simulink model "Non_isolated_Buck_Boost_Converter_w_NonIdealities"  (R2021a)
settings: Solver=VariableStepAuto  StartTime=0.0  StopTime=0.1  RelTol=1e-3
libraries: spsSeriesRLCBranchLib x5, spsCurrentMeasurementLib x4, spsVoltageMeasurementLib x3, spsDiodeLib x1, spsMosfetLib x1, spsDCVoltageSourceLib x1, spspowerguiLib x1
settings Model: Creator=EREN-PC  LastModifiedBy=EREN-PC

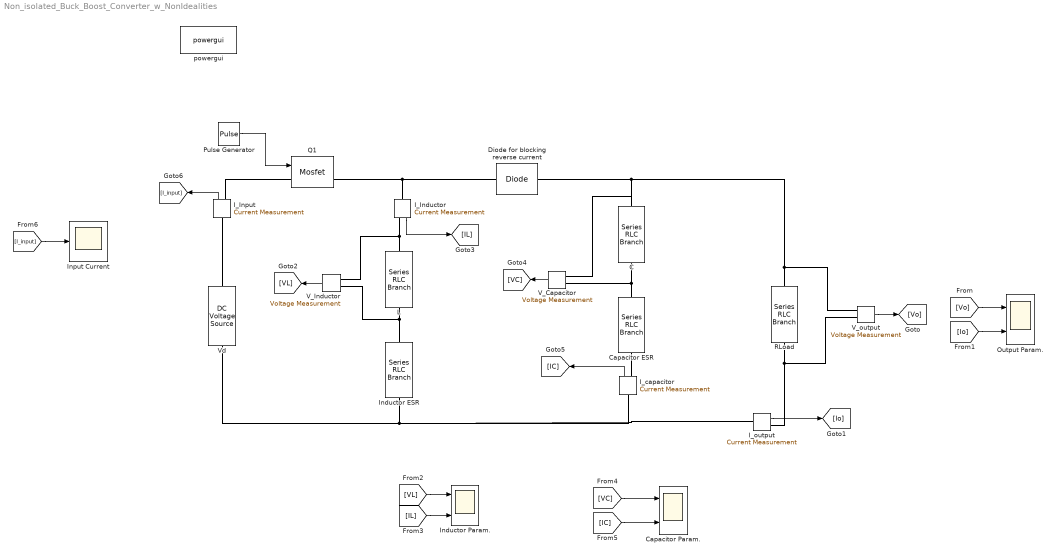
== system Non_isolated_Buck_Boost_Converter_w_NonIdealities ==
  C : spsSeriesRLCBranchLib/Series RLC Branch  LConnTagsString=__new0  RConnTagsString=__new0  BranchType=C  Resistance=1  Inductance=1e-3  SetiL0=off  InitialCurrent=0  Capacitance=1e-3  Setx0=off  InitialVoltage=0  Measurements=None
  Capacitor ESR : spsSeriesRLCBranchLib/Series RLC Branch  LConnTagsString=__new0  RConnTagsString=__new0  BranchType=R  Resistance=12e-3  Inductance=1e-3  SetiL0=off  InitialCurrent=0  Capacitance=1e-6  Setx0=off  InitialVoltage=0  Measurements=None
  Capacitor Param. : Scope  NumInputPorts=2
  Diode for blocking reverse current : spsDiodeLib/Diode  Ron=0.001  Lon=0  Vf=0.45  IC=0  UseSnubber=0  Rs=500  Cs=250e-9  Measurements=off
  I_Inductor : spsCurrentMeasurementLib/Current Measurement  PhasorSimulation=off  OutputType=Complex  PSBequivalent=0
  I_Input : spsCurrentMeasurementLib/Current Measurement  PhasorSimulation=off  OutputType=Complex  PSBequivalent=0
  I_capacitor : spsCurrentMeasurementLib/Current Measurement  PhasorSimulation=off  OutputType=Complex  PSBequivalent=0
  I_output : spsCurrentMeasurementLib/Current Measurement  PhasorSimulation=off  OutputType=Complex  PSBequivalent=0
  Inductor ESR : spsSeriesRLCBranchLib/Series RLC Branch  LConnTagsString=__new0  RConnTagsString=__new0  BranchType=R  Resistance=0.494  Inductance=1e-3  SetiL0=off  InitialCurrent=0  Capacitance=1e-6  Setx0=off  InitialVoltage=0  Measurements=None
  Inductor Param. : Scope  NumInputPorts=2
  Input Current : Scope
  L : spsSeriesRLCBranchLib/Series RLC Branch  LConnTagsString=__new0  RConnTagsString=__new0  BranchType=L  Resistance=0.494  Inductance=2.2e-3  SetiL0=off  InitialCurrent=0  Capacitance=1e-6  Setx0=off  InitialVoltage=0  Measurements=None
  Output Param. : Scope  NumInputPorts=2
  Pulse Generator : DiscretePulseGenerator  PulseType=Time based  Period=20e-6  PulseWidth=52
  Q1 : spsMosfetLib/Mosfet  Ron=60e-3  Lon=0  Rd=25e-3  Vfd=0  IC=0  Rs=1e5  Cs=inf  Measurements=on
  RLoad : spsSeriesRLCBranchLib/Series RLC Branch  LConnTagsString=__new0  RConnTagsString=__new0  BranchType=R  Resistance=6  Inductance=1e-3  SetiL0=off  InitialCurrent=0  Capacitance=1e-6  Setx0=off  InitialVoltage=0  Measurements=None
  V_Capacitor : spsVoltageMeasurementLib/Voltage Measurement  PhasorSimulation=off  OutputType=Complex  PSBequivalent=0
  V_Inductor : spsVoltageMeasurementLib/Voltage Measurement  PhasorSimulation=off  OutputType=Complex  PSBequivalent=0
  V_output : spsVoltageMeasurementLib/Voltage Measurement  PhasorSimulation=off  OutputType=Complex  PSBequivalent=0
  Vd : spsDCVoltageSourceLib/DC Voltage Source  Amplitude=16  Measurements=None
  powergui : spspowerguiLib/powergui  Priority=1  SimulationMode=Continuous  SampleTime=50e-6  frequency=60  Iterations=50  frequencyindice=0  Pbase=100e6  ErrMax=1e-4  UnitsV=kV  UnitsW=MW  buscounter=0  FunctionMessages=off  echomessages=off  EnableUseOfTLC=off  CurrentSourceSwitches=off  DisableSnubberDevices=off  DisableRonSwitches=off  DisableVfSwitches=off  DisplayEquations=off  AutomaticDiscreteSolvers=off  SolverType=Tustin/Backward Euler (TBE)  Interpol=off  ExternalGateDelay=off  methode=off  Ts=100  x0status=blocks  SPID=on  SwTol=0  HookPort=off  NonlinearTolerance=1e-4  nMaxIteration=100  ContinueOnMaxIteration=off  RestoreLinks=warning  ResistiveCurrentMeasurement=off  Frange=[0:2:500]  Ylog=off  Xlog=on  ShowGrid=off  save=off  variable=ZData  structure=0  ZoomFFT=off  StartTime=0.0  cycles=1  DisplayStyle=1  fundamental=60  FreqAxis=off  MaxFrequency=1000  frequencyindicesteady=1  RmsSteady=1  display=off
  wires:
  V_output/1 -> [Vo]
  [Vo] -> Output Param./1
  I_output/1 -> [Io]
  [Io] -> Output Param./2
  V_Inductor/1 -> [VL]
  [VL] -> Inductor Param./1
  I_Inductor/1 -> [IL]
  [IL] -> Inductor Param./2
  V_Capacitor/1 -> [VC]
  [VC] -> Capacitor Param./1
  I_capacitor/1 -> [IC]
  [IC] -> Capacitor Param./2
  Pulse Generator/1 -> Q1/1
  I_Input/1 -> [I_input]
  [I_input] -> Input Current/1
  connections:
  Inductor ESR/RConn1 -- I_capacitor/LConn1 -- I_output/LConn1 -- Vd/LConn1
  Q1/RConn1 -- I_Inductor/LConn1 -- Diode for blocking reverse current/RConn1
  L/LConn1 -- Inductor ESR/LConn1 -- V_Inductor/LConn2
  Capacitor ESR/LConn1 -- V_Capacitor/LConn1 -- C/RConn1
  Diode for blocking reverse current/LConn1 -- V_Capacitor/LConn2 -- C/LConn1 -- V_output/LConn2 -- RLoad/LConn1
  V_output/LConn1 -- I_output/RConn1 -- RLoad/RConn1
  V_Inductor/LConn1 -- I_Inductor/RConn1 -- L/RConn1
  I_capacitor/RConn1 -- Capacitor ESR/RConn1
  I_Input/LConn1 -- Vd/RConn1
  I_Input/RConn1 -- Q1/LConn1
